simulink model "task_2_sim"  (R2022b)
settings: Solver=VariableStepAuto  StartTime=0.0  StopTime=10.0  RelTol=1e-3
model workspace (MAT data in the model file):
  C0 = [1  0  0  0  0  0; 0  1  0  0  0  0; 0  0  1  0  0  0; 0  0  0  1  0  0; 0  0  0  0  1  0; 0  0  0  0  0  1]
  D0 = [0  0; 0  0; 0  0; 0  0; 0  0; 0  0]
values from neighbouring files (symbols this model uses):
  A = [0 0 0 1 0 0 ... (first row only)    [buildStateSpaceModel.m]
  B = [0 0 ... (first row only)    [buildStateSpaceModel.m]
  C = [1 0 0 0 0 0 ... (first row only)    [buildStateSpaceModel.m]
  K2_1 = getLQRController(A, B, Q, R)    [task2.m]
  K2_2 = getLQRController(A, B, 50*Q, R)    [task2.m]
  x0 = [0.2; -0.1; 0.15; -1; 0.8; 0]    [buildStateSpaceModel.m]
settings Model: Creator=小灰  LastModifiedBy=小灰

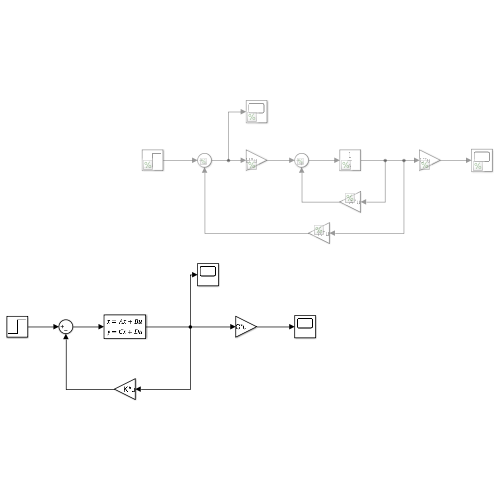
[thumbnail: Simulink's stored preview of the top-level diagram]
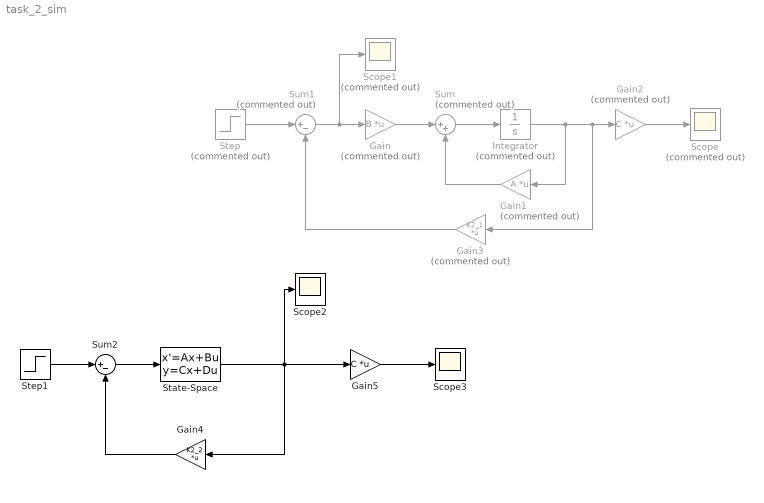
== system task_2_sim ==
  Gain : Gain  Commented=on  Gain=B  Multiplication=Matrix(K*u)
  Gain1 : Gain  Commented=on  Gain=A  Multiplication=Matrix(K*u)
  Gain2 : Gain  Commented=on  Gain=C  Multiplication=Matrix(K*u)
  Gain3 : Gain  Commented=on  Gain=K2_1  Multiplication=Matrix(K*u)
  Gain4 : Gain  Gain=K2_2  Multiplication=Matrix(K*u)
  Gain5 : Gain  Gain=C  Multiplication=Matrix(K*u)
  Integrator : Integrator  Commented=on
  Scope : Scope  Commented=on
  Scope1 : Scope  Commented=on
  Scope2 : Scope
  Scope3 : Scope
  State-Space : StateSpace  A=A  B=B  C=C0  D=D0  InitialCondition=x0  ParameterTunability=Unconstrained
  Step : Step  Commented=on  SampleTime=0
  Step1 : Step  Before=[0, 0]  After=[1, 1]  SampleTime=0
  Sum : Sum  Commented=on  Inputs=|++
  Sum1 : Sum  Commented=on  Inputs=|+-
  Sum2 : Sum  Inputs=|+-
  wires:
  Integrator/1 -> Gain1/1, Gain3/1, Gain2/1
  Sum/1 -> Integrator/1
  Step/1 -> Sum1/1
  Gain2/1 -> Scope/1
  Gain1/1 -> Sum/2
  Sum1/1 -> Scope1/1, Gain/1
  Gain/1 -> Sum/1
  Gain3/1 -> Sum1/2
  State-Space/1 -> Gain5/1, Gain4/1, Scope2/1
  Gain4/1 -> Sum2/2
  Sum2/1 -> State-Space/1
  Step1/1 -> Sum2/1
  Gain5/1 -> Scope3/1
